simulink model "Sistema"  (R2023a)
settings: Solver=VariableStepAuto  StartTime=0.0  StopTime=100  FixedStep=1E-3  MaxStep=1e-3  RelTol=1e-6
libraries: slpidlib x1
settings Model: Creator=Bricia Arellano  LastModifiedBy=Bricia Arellano
settings DataIOCC: ReturnWorkspaceOutputs=off  TimeSaveName=t
settings DebuggingCC: AlgebraicLoopMsg=none  ArtificialAlgebraicLoopMsg=none  MaxConsecutiveZCsMsg=none  ModelReferenceExtraNoncontSigs=none  OperatingPointInterfaceChecksumMismatchMsg=none

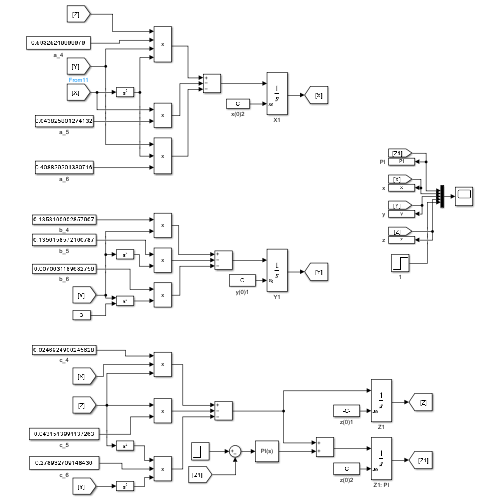
[thumbnail: Simulink's stored preview of the top-level diagram]
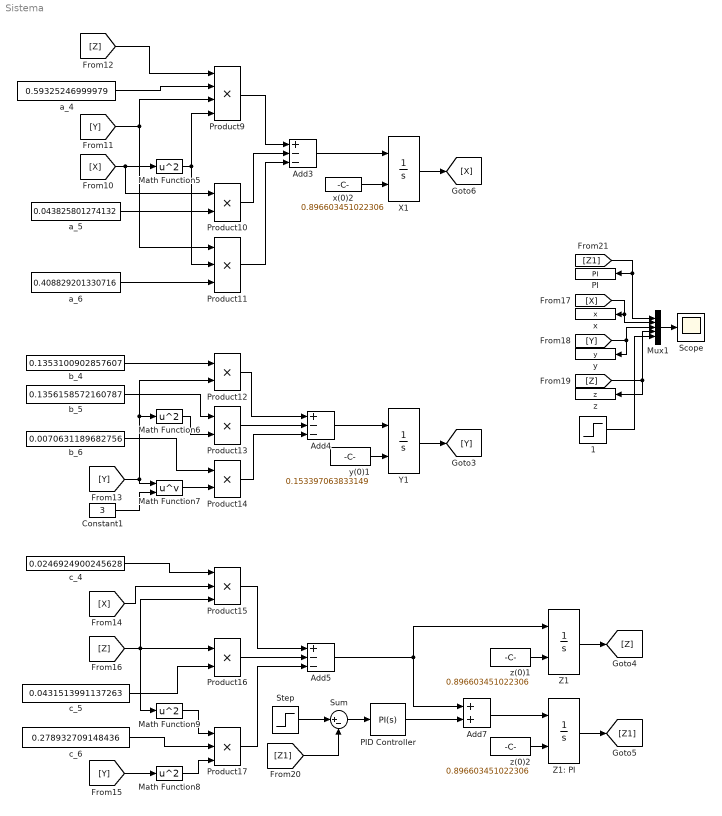
== system Sistema ==
  1 : Step  Time=0  SampleTime=0
  Add3 : Sum  Inputs=+--
  Add4 : Sum  Inputs=+--
  Add5 : Sum  Inputs=+--
  Add7 : Sum
  Constant1 : Constant  Value=3
  Math Function{5..6,8..9} (4 alike) : Math  Operator=square
  Math Function7 : Math  Operator=pow
  Mux1 : Mux  Inputs=5
  PI : ToWorkspace  VariableName=PI  SampleTime=-1
  PID Controller : slpidlib/PID Controller  Controller=PI  Form=Parallel  TimeDomain=Continuous-time  UseExternalTs=off  SampleTime=-1  IntegratorMethod=Forward Euler  FilterMethod=Forward Euler  ControllerParametersSource=internal  P=0.9999  I=0.002  UseKiTs=off  D=0  N=100  UseFilter=on  TunerSelectOption=Transfer Function Based (PID Tuner App)  InitialConditionSource=internal  InitialConditionForIntegrator=0  InitialConditionForFilter=0  DifferentiatorICPrevScaledInput=0  ExternalReset=none  TrackingMode=off  Kt=1  LimitOutput=off  SatLimitsSource=internal  UpperSaturationLimit=inf  LowerSaturationLimit=-inf  LinearizeAsGain=on  AntiWindupMode=none  Kb=1  LimitIntegrator=off  UpperIntegratorSaturationLimit=inf  LowerIntegratorSaturationLimit=-inf  POutMin=[]  POutMax=[]  IOutMin=[]  IOutMax=[]  DOutMin=[]  DOutMax=[]  NOutMin=[]  NOutMax=[]  SumOutMin=[]  SumOutMax=[]  SaturationOutMin=[]  SaturationOutMax=[]  PParamMin=[]  PParamMax=[]  IParamMin=[]  IParamMax=[]  DParamMin=[]  DParamMax=[]  NParamMin=[]  NParamMax=[]  KbParamMin=[]  KbParamMax=[]  KtParamMin=[]  KtParamMax=[]  KbOutMin=[]  KbOutMax=[]  KtOutMin=[]  KtOutMax=[]  IntegratorOutMin=[]  IntegratorOutMax=[]  FilterOutMin=[]  FilterOutMax=[]  SumI1OutMin=[]  SumI1OutMax=[]  SumI2OutMin=[]  SumI2OutMax=[]  SumI3OutMin=[]  SumI3OutMax=[]  SumI4OutMin=[]  SumI4OutMax=[]  SumDOutMin=[]  SumDOutMax=[]  DifferentiatorOutMin=[]  DifferentiatorOutMax=[]  FilterDiffOutCoefMin=[]  FilterDiffOutCoefMax=[]  ReciprocalOutMin=[]  ReciprocalOutMax=[]  SumDenOutMin=[]  SumDenOutMax=[]  SumNumOutMin=[]  SumNumOutMax=[]  DivideOutMin=[]  DivideOutMax=[]  UdiffTsProdOutMin=[]  UdiffTsProdOutMax=[]  NTsProdOutMin=[]  NTsProdOutMax=[]  UintegralTsProdOutMin=[]  UintegralTsProdOutMax=[]  UngainTsProdOutMin=[]  UngainTsProdOutMax=[]  ClampingZeroOutDataTypeStr=Inherit: Inherit via back propagation  ClampingZeroOutMin=[]  ClampingZeroOutMax=[]  FilterDenConstantOutDataTypeStr=Inherit: Inherit via back propagation  FilterDenConstantOutMin=[]  FilterDenConstantOutMax=[]  PCopyOutDataTypeStr=Inherit: Inherit via back propagation  PCopyOutMin=[]  PCopyOutMax=[]  NCopyOutDataTypeStr=Inherit: Inherit via back propagation  NCopyOutMin=[]  NCopyOutMax=[]  IntegratorContinuousStateAttributes=''  IntegratorStateMustResolveToSignalObject=off  IntegratorRTWStateStorageClass=Auto  FilterContinuousStateAttributes=''  FilterStateMustResolveToSignalObject=off  FilterRTWStateStorageClass=Auto  ParallelPVariant=InternalParameters  IdealPVariant=Disabled  IVariant=InternalParameters  DVariant=Disabled  IntegratorVariant=Continuous  SatVariant=Disabled  AWVariant=Passthrough  PCopyVariant=Disabled  TRVariant=Disabled  FdbkBlocksVariant=Forward  IdealPFdbkVariant=Disabled  SatFdbkVariant=Disabled  DerivativeFilterVariant=Disabled  NVariant=Disabled  NCopyVariant=Disabled_SignalSpec  FilterICVariant=Disabled  IntegratorICVariant=InternalICs  ExternalResetVariant=Disabled  TRSumVariant=Passthrough  SumFdbkVariant=Disabled  SumVariant=Sum_PI  TsampFilterVariant=InternalTs  TsampNgainVariant=Passthrough  TsampIntegralVariant=Disabled_SignalSpec  ExternalSaturationOutDataTypeStr=Inherit: Same as second input
  Product{10,12..14,16} (5 alike) : Product
  Product11 : Product  Inputs=3
  Product15 : Product  Inputs=3
  Product17 : Product  Inputs=3
  Product9 : Product  Inputs=4
  Scope : Scope
  Step : Step  Time=0  SampleTime=0
  Sum : Sum  Inputs=|+-
  X1 : Integrator  InitialConditionSource=external
  Y1 : Integrator  InitialConditionSource=external
  Z1 : Integrator  InitialConditionSource=external
  Z1: PI : Integrator  InitialConditionSource=external
  a_4 : Constant  Value=0.59325246999979
  a_5 : Constant  Value=0.043825801274132
  a_6 : Constant  Value=0.408829201330716
  b_4 : Constant  Value=0.1353100902857607
  b_5 : Constant  Value=0.1356158572160787
  b_6 : Constant  Value=0.0070631189682756
  c_4 : Constant  Value=0.0246924900245628
  c_5 : Constant  Value=0.0431513991137263
  c_6 : Constant  Value=0.278932709148436
  x : ToWorkspace  VariableName=x  SampleTime=-1
  x(0)2 : Constant  Value=0.896603451022306
  y : ToWorkspace  VariableName=y  SampleTime=-1
  y(0)1 : Constant  Value=0.153397063833149
  z : ToWorkspace  VariableName=z  SampleTime=-1
  z(0)1 : Constant  Value=0.896603451022306
  z(0)2 : Constant  Value=0.896603451022306
  wires:
  z(0)1/1 -> Z1/2
  Y1/1 -> [Y]
  Product14/1 -> Add4/3
  Product17/1 -> Add5/3
  [X] -> Product15/2
  Mux1/1 -> Scope/1
  Math Function8/1 -> Product17/3
  Product16/1 -> Add5/2
  Math Function7/1 -> Product14/2
  Product11/1 -> Add3/3
  Math Function9/1 -> Product17/1
  [Y] -> Math Function7/1, Math Function6/1, Product12/2
  Add4/1 -> Y1/1
  a_6/1 -> Product11/3
  b_6/1 -> Product14/1
  Product12/1 -> Add4/1
  a_5/1 -> Product10/2
  Z1/1 -> [Z]
  c_5/1 -> Product16/2
  Product10/1 -> Add3/2
  Product13/1 -> Add4/2
  b_5/1 -> Product13/1
  y(0)1/1 -> Y1/2
  b_4/1 -> Product12/1
  [Y] -> Product11/1, Product9/3
  Product15/1 -> Add5/1
  Product9/1 -> Add3/1
  Math Function5/1 -> Product11/2, Product9/4
  Math Function6/1 -> Product13/2
  Constant1/1 -> Math Function7/2
  c_6/1 -> Product17/2
  c_4/1 -> Product15/1
  [X] -> Math Function5/1, Product10/1
  [Y] -> Math Function8/1
  a_4/1 -> Product9/2
  [Z] -> Product9/1
  [Z] -> Product16/1, Product15/3, Math Function9/1
  Sum/1 -> PID Controller/1
  Add7/1 -> Z1: PI/1
  X1/1 -> [X]
  x(0)2/1 -> X1/2
  Step/1 -> Sum/1
  [Z1] -> Sum/2
  [X] -> x/1, Mux1/2
  [Y] -> y/1, Mux1/3
  [Z] -> z/1, Mux1/4
  Z1: PI/1 -> [Z1]
  [Z1] -> PI/1, Mux1/1
  Add5/1 -> Add7/1, Z1/1
  PID Controller/1 -> Add7/2
  Add3/1 -> X1/1
  z(0)2/1 -> Z1: PI/2
  1/1 -> Mux1/5
